simulink model "lqr"  (R2017a)
settings: Solver=VariableStepAuto  StartTime=0.0  StopTime=5  RelTol=1e-3
values from neighbouring files (symbols this model uses):
  DCgain7 = D7d + C7cl*inv(eye(3)-A7cl)*B7d    [q13.m]    (also in q5.m; q5_reduced.m)
  h7 = 0.08    [q13.m]    (also in q5.m = 0.006; q5_reduced.m)
undefined symbols (not defined in the file or in its folder): A7d, B7d, C7d, D7d, K7
settings Model: Creator=Aleksandra  LastModifiedBy=Aleksandra

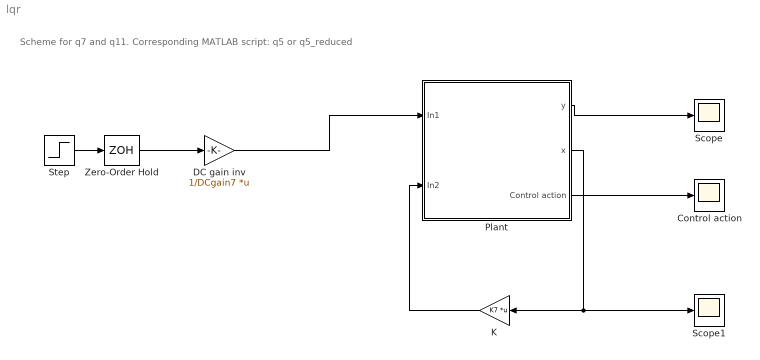
== system lqr ==
  note: Scheme for q7 and q11.
      | Corresponding MATLAB script: q5 or q5_reduced
  Control action : Scope
  DC gain inv : Gain  Gain=1/DCgain7  Multiplication=Matrix(K*u)
  K : Gain  Gain=K7  Multiplication=Matrix(K*u)
  Plant : Subsystem
  Scope : Scope
  Scope1 : Scope
  Step : Step  Time=0  SampleTime=0
  Zero-Order Hold : ZeroOrderHold  SampleTime=h7
  wires:
  K/1 -> Plant/2(In2)
  Plant/1(y) -> Scope/1
  Plant/2(x) -> Scope1/1, K/1
  Step/1 -> Zero-Order Hold/1
  Zero-Order Hold/1 -> DC gain inv/1
  DC gain inv/1 -> Plant/1(In1)
  Plant/3(Control action) -> Control action/1

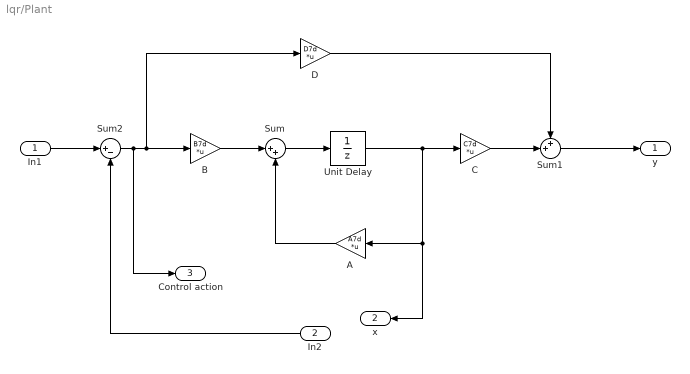
== system lqr/Plant ==
  In1 : Inport
  In2 : Inport  Port=2
  A : Gain  Gain=A7d  Multiplication=Matrix(K*u)
  B : Gain  Gain=B7d  Multiplication=Matrix(K*u)
  C : Gain  Gain=C7d  Multiplication=Matrix(K*u)
  D : Gain  Gain=D7d  Multiplication=Matrix(K*u)
  Sum : Sum  Inputs=|++
  Sum1 : Sum  Inputs=++|
  Sum2 : Sum  Inputs=|+-
  Unit Delay : UnitDelay  SampleTime=-1
  y : Outport
  x : Outport  Port=2
  Control action : Outport  Port=3
  wires:
  Sum/1 -> Unit Delay/1
  A/1 -> Sum/2
  D/1 -> Sum1/1
  C/1 -> Sum1/2
  Sum1/1 -> y/1
  B/1 -> Sum/1
  Sum2/1 -> Control action/1, D/1, B/1
  Unit Delay/1 -> x/1, A/1, C/1
  In2/1 -> Sum2/2
  In1/1 -> Sum2/1
